simulink model "abishek_hariharan_hw1"  (Simulink 7.8)
settings: Solver=ode45  StartTime=0.0  StopTime=40.0  RelTol=1e-3
settings Model: Creator=abishekh  LastModifiedBy=abishekh

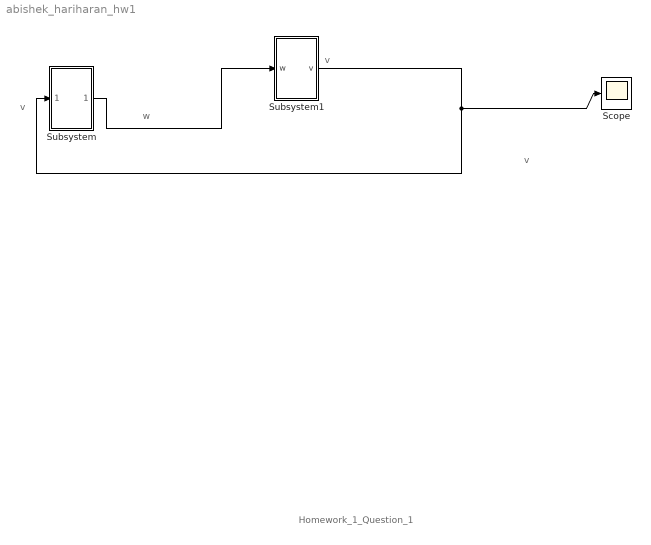
== system abishek_hariharan_hw1 ==
  note: Homework_1_Question_1
  note: v
  note: v
  note: v
  note: w
  Scope : Scope
      settings: MaxDataPoints=0
  Subsystem : Subsystem
  Subsystem1 : Subsystem
  wires:
  Subsystem/1(Out1) -> Subsystem1/1(w)
  Subsystem1/1(v) -> Subsystem/1(In1), Scope/1

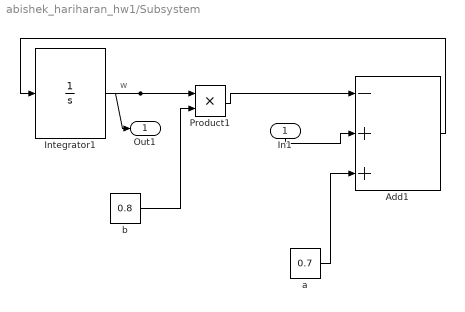
== system abishek_hariharan_hw1/Subsystem ==
  note: w
  In1 : Inport
  Add1 : Sum  Inputs=-++
  Integrator1 : Integrator
  Product1 : Product  RndMeth=Zero
  a : Constant  Value=0.7
  b : Constant  Value=0.8
  Out1 : Outport
  wires:
  Product1/1 -> Add1/1
  b/1 -> Product1/2
  Integrator1/1 -> Product1/1, Out1/1
  Add1/1 -> Integrator1/1
  a/1 -> Add1/3
  In1/1 -> Add1/2

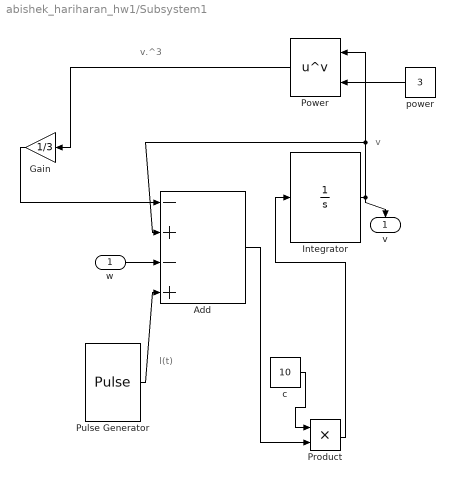
== system abishek_hariharan_hw1/Subsystem1 ==
  note: v
  note: l(t)
  note: v.^3
  w : Inport
  Add : Sum  Inputs=-+-+
  Gain : Gain  Gain=1/3
  Integrator : Integrator
  Power : Math  Operator=pow  SaturateOnIntegerOverflow=on
  Product : Product  RndMeth=Zero
  Pulse Generator : DiscretePulseGenerator  PulseType=Time based  Amplitude=0.4  Period=1  PulseWidth=99.9
  c : Constant  Value=10
  power : Constant  Value=3
  v : Outport
  wires:
  Integrator/1 -> Add/2, Power/1, v/1
  Pulse Generator/1 -> Add/4
  Add/1 -> Product/2
  power/1 -> Power/2
  Power/1 -> Gain/1
  Gain/1 -> Add/1
  Product/1 -> Integrator/1
  c/1 -> Product/1
  w/1 -> Add/3
